simulink model "boat"  (Simulink 7.9)
settings: Solver=ode45  StartTime=0.0  StopTime=10.0  RelTol=1e-3
values from neighbouring files (symbols this model uses):
  friX = 3    [initial_parameters.m]
  friY = 8    [initial_parameters.m]
  I = 1/12*M*((2*ry1)^2 + (2*rx1)^2)    (= 7.46230507536)    [initial_parameters.m]
  M = 80*lbtokg    (= 36.28736)    [initial_parameters.m]
  rx1 = -69*intom/2 + 6*intom    (= -0.7239)    [initial_parameters.m]
  ry1 = -12*intom    (= -0.3048)    [initial_parameters.m]
  ry2 = 12*intom    (= 0.3048)    [initial_parameters.m]
settings Model: Creator=darsan13  LastModifiedBy=Darsan
settings DataIOCC: SignalLoggingSaveFormat=Dataset
settings OptimizationCC: ExpressionDepthLimit=128
settings DebuggingCC: StateNameClashWarn=none
settings CodeAppCC: CustomSymbolStrType=$N$R$M_T

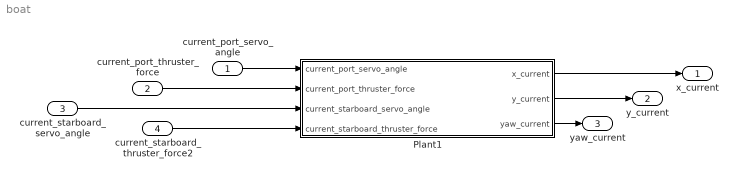
== system boat ==
  current_port_servo_angle : Inport
  current_port_thruster_force : Inport  Port=2
  current_starboard_servo_angle : Inport  Port=3
  current_starboard_thruster_force2 : Inport  Port=4
  Plant1 : Subsystem  mask{rx1=rx1, ry1=ry1, ry2=ry2, M=M, I=I, friX=friX, friY=friY}
  x_current : Outport
  y_current : Outport  Port=2
  yaw_current : Outport  Port=3
  wires:
  current_port_thruster_force/1 -> Plant1/2(current_port_thruster_force)
  current_port_servo_angle/1 -> Plant1/1(current_port_servo_angle)
  current_starboard_servo_angle/1 -> Plant1/3(current_starboard_servo_angle)
  current_starboard_thruster_force2/1 -> Plant1/4(current_starboard_thruster_force)
  Plant1/3(yaw_current) -> yaw_current/1
  Plant1/2(y_current) -> y_current/1
  Plant1/1(x_current) -> x_current/1

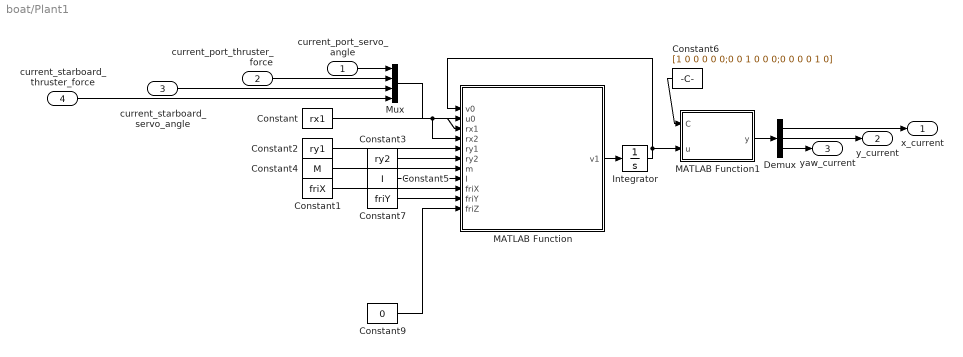
== system boat/Plant1 ==
  current_port_servo_angle : Inport
  current_port_thruster_force : Inport  Port=2
  current_starboard_servo_angle : Inport  Port=3
  current_starboard_thruster_force : Inport  Port=4
  Constant : Constant  Value=rx1
  Constant1 : Constant  Value=friX
  Constant2 : Constant  Value=ry1
  Constant3 : Constant  Value=ry2
  Constant4 : Constant  Value=M
  Constant5 : Constant  Value=I
  Constant6 : Constant  Value=[1 0 0 0 0 0;0 0 1 0 0 0;0 0 0 0 1 0]
  Constant7 : Constant  Value=friY
  Constant9 : Constant  Value=0
  Demux : Demux  Outputs=3
  Integrator : Integrator  InitialCondition=[0 0 0 0 0 0]
  MATLAB Function : MATLAB Function  TreatAsAtomicUnit=on
  MATLAB Function1 : MATLAB Function  TreatAsAtomicUnit=on
  Mux : Mux
  x_current : Outport
  y_current : Outport  Port=2
  yaw_current : Outport  Port=3
  wires:
  Constant/1 -> MATLAB Function/3(rx1), MATLAB Function/4(rx2)
  Constant2/1 -> MATLAB Function/5(ry1)
  Constant3/1 -> MATLAB Function/6(ry2)
  Constant4/1 -> MATLAB Function/7(m)
  Constant5/1 -> MATLAB Function/8(I)
  MATLAB Function/1(v1) -> Integrator/1
  Integrator/1 -> MATLAB Function/1(v0), MATLAB Function1/2(u)
  Constant6/1 -> MATLAB Function1/1(C)
  MATLAB Function1/1(y) -> Demux/1
  Demux/2 -> y_current/1
  Demux/3 -> yaw_current/1
  Demux/1 -> x_current/1
  current_port_servo_angle/1 -> Mux/1
  current_port_thruster_force/1 -> Mux/2
  current_starboard_servo_angle/1 -> Mux/3
  current_starboard_thruster_force/1 -> Mux/4
  Mux/1 -> MATLAB Function/2(u0)
  Constant1/1 -> MATLAB Function/9(friX)
  Constant7/1 -> MATLAB Function/10(friY)
  Constant9/1 -> MATLAB Function/11(friZ)

== matlab function Plant1/MATLAB Function ==
  data: v0 input double; v1 output double; u0 input double; rx1 input double; rx2 input double; ry1 input double; ry2 input double; m input double; I input double; friX input double; friY input double; friZ input double
function v1   = boatDynamics(v0, u0, rx1, rx2, ry1, ry2, m, I, friX, friY, friZ)

    % %%%%%%%%%%%%%%%%%%%%%%%%%%%%%%%%%%%%%%%%%%%% %
    %    v = [x...          %    u = [theta1...    %
    %        x_dot...       %        f1...         %
    %        y...           %        theta2...     %
    %        y_dot...       %        f2]           %
    %        theta...       %                      %
    %        theta_dot];    %                      %
    % %%%%%%%%%%%%%%%%%%%%%%%%%%%%%%%%%%%%%%%%%%%% %
    
    v11 = v0(2);
    v12 = u0(2)/m*cosd(u0(1)+v0(5)) + u0(4)/m*cosd(u0(3)+v0(5)) - friX*v0(2)*(cosd(v0(5))+sind(v0(5)));
    v13 = v0(4);
    v14 = u0(2)/m*sind(u0(1)+v0(5)) + u0(4)/m*sind(u0(3)+v0(5)) - friY*v0(4)*(-sind(v0(5))+cosd(v0(5)));
    v15 = v0(6);
    v16 = rx1/I*u0(2)*sind(u0(1)) - ry1/I*u0(2)*cosd(u0(1)) + rx2/I*u0(4)*sind(u0(3)) - ry2/I*u0(4)*cosd(u0(3)) - friZ*v0(6);
   
    v1 = [v11;v12;v13;v14;v15;v16];
    
    
end

== matlab function Plant1/MATLAB Function1 ==
  data: C input double; u input double; y output double
function y = fcn(C,u)
%#codegen

y = C*u;
